simulink model "Stiffness"  (R2023b)
settings: Solver=ode4  StartTime=0.0  StopTime=25  FixedStep=0.1  RelTol=1e-3
values from neighbouring files (symbols this model uses):
  A = A_values(A_index)    [Part_1_Final.m]
  b = b_values(b_index)    [Part_1_Final.m]
  J = J_values(J_index)    [Part_1_Final.m]
  w_0 = w_0_values(w0_index)    [Part_1_Final.m]
settings Model: Creator=oscar  LastModifiedBy=oscar

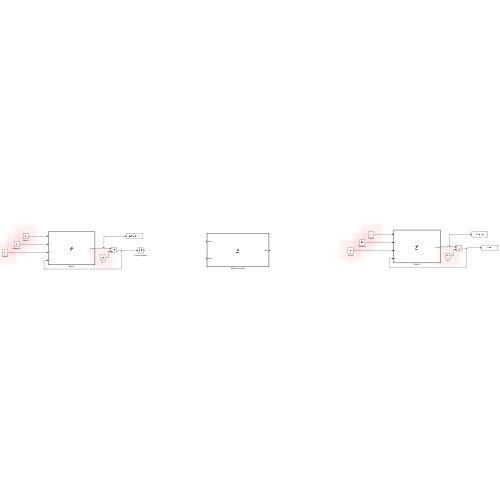
[thumbnail: Simulink's stored preview of the top-level diagram]
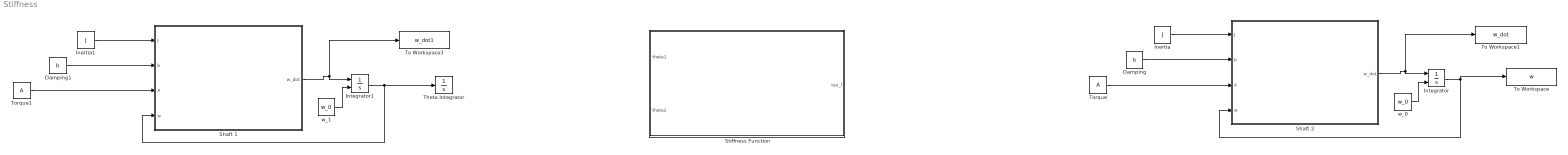
== system Stiffness ==
  Damping : Constant  Value=b
  Damping1 : Constant  Value=b
  Inertia : Constant  Value=J
  Inertia1 : Constant  Value=J
  Integrator : Integrator  InitialConditionSource=external  LimitOutput=on  UpperSaturationLimit=1000
  Integrator1 : Integrator  InitialConditionSource=external  LimitOutput=on  UpperSaturationLimit=1000
  Shaft 1 : MATLAB Function  TreatAsAtomicUnit=on
  Shaft 2 : MATLAB Function  TreatAsAtomicUnit=on
  Stiffness Function : MATLAB Function  TreatAsAtomicUnit=on
  Theta Integrator : Integrator  LimitOutput=on  UpperSaturationLimit=1000
  To Workspace : ToWorkspace  VariableName=w  SaveFormat=Structure With Time  SampleTime=-1
  To Workspace1 : ToWorkspace  VariableName=w_dot  SaveFormat=Structure With Time  SampleTime=-1
  To Workspace3 : ToWorkspace  VariableName=w_dot1  SaveFormat=Structure With Time  SampleTime=-1
  Torque : Constant  Value=A
  Torque1 : Constant  Value=A
  w_0 : Constant  Value=w_0
  w_1 : Constant  Value=w_0
  wires:
  Shaft 2/1(w_dot) -> To Workspace1/1, Integrator/1
  Inertia/1 -> Shaft 2/1(J)
  Damping/1 -> Shaft 2/2(b)
  Torque/1 -> Shaft 2/3(A)
  Integrator/1 -> To Workspace/1, Shaft 2/4(w)
  w_0/1 -> Integrator/2
  w_1/1 -> Integrator1/2
  Torque1/1 -> Shaft 1/3(A)
  Damping1/1 -> Shaft 1/2(b)
  Inertia1/1 -> Shaft 1/1(J)
  Integrator1/1 -> Theta Integrator/1, Shaft 1/4(w)
  Shaft 1/1(w_dot) -> To Workspace3/1, Integrator1/1

== matlab function Stiffness/Shaft 1 ==
  data: J input; w_dot output; b input; A input; w input
function w_dot = fcn(J, b, A, w)

w_dot = (1/J)*(A-(b*w));

end

== matlab function Stiffness/Shaft 2 ==
  data: J input; w_dot output; b input; A input; w input
function w_dot = fcn(J, b, A, w)

w_dot = (1/J)*(A-(b*w));

end

== matlab function Stiffness/Stiffness Function ==
  data: theta1 input; tau_l output; theta2 input
function tau_l = fcn(theta1, theta2)

y = u;
